simulink model "CHEM_FULL_BENCHMARK"  (R2019a)
settings: Solver=FixedStepAuto  StartTime=0.0  StopTime=app.SimuTime  FixedStep=Te  RelTol=1e-3  EnableMultiTasking=on
values from neighbouring files (symbols this model uses):
  A1 = 0.0154    [INIT_FULL.m]    (also in run.m)
  A2 = 0.0154    [INIT_FULL.m]    (also in run.m)
  app = interface    [INIT_FULL.m]    (also in run.m)
  Cvb = 1.5938*1e-4    (= 0.00015938)    [INIT_FULL.m]    (also in run.m)
  Cvo = 1.59640*1e-4    (= 0.00015964)    [INIT_FULL.m]    (also in run.m)
  g = 9.81    [INIT_FULL.m]    (also in run.m)
  h1c = 0.5    [INIT_FULL.m]    (also in run.m)
  h1c_0 = 0    [INIT_FULL.m]    (also in run.m)
  h1max = 0.6    [INIT_FULL.m]    (also in run.m)
  h2c_0 = 0    [INIT_FULL.m]    (also in Variables_Update.m = app.InitialwaterlevelinT206EditField.Value; run.m)
  h2c_max = 0.11    [INIT_FULL.m]    (also in run.m)
  h2c_min = 0.09    [INIT_FULL.m]    (also in run.m)
  h2max = 0.6    [INIT_FULL.m]    (also in run.m)
  Ki = 5*1e-6    (= 5e-06)    [INIT_FULL.m]    (also in run.m)
  Kp = 1e-3    (= 0.001)    [INIT_FULL.m]    (also in run.m)
  Patm = 101325    [INIT_FULL.m]    (also in run.m)
  Qf1 = 1e-4    (= 0.0001)    [INIT_FULL.m]    (also in Variables_Update.m = app.FlowleakfromT1m3sEditField.Value; run.m)
  Qf2 = 1e-4    (= 0.0001)    [INIT_FULL.m]    (also in Variables_Update.m = app.FlowleakfromT2m3sEditField.Value; run.m)
  Qof1 = 1e-4    (= 0.0001)    [INIT_FULL.m]    (also in Variables_Update.m = app.OverflowrateinT1m3sEditField.Value; run.m)
  Qpmax = 1e-2    (= 0.01)    [INIT_FULL.m]    (also in run.m)
  rate_noise_mQp = 0.01*1e-5    (= 1e-07)    [INIT_FULL.m]    (also in run.m)
  rate_noise_mUp = 0.01*1e-5    (= 1e-07)    [INIT_FULL.m]    (also in run.m)
  rate_noise_my1 = 0.5*0.001    (= 0.0005)    [INIT_FULL.m]    (also in run.m)
  rate_noise_my2 = 0.3*0.001    (= 0.0003)    [INIT_FULL.m]    (also in run.m)
  ro = 1000    [INIT_FULL.m]    (also in run.m)
  seed = randi(10000000)    [INIT_FULL.m]    (also in run.m)
  Te = 1    [INIT_FULL.m]    (also in run.m)
  yo = 0    [INIT_FULL.m]    (also in run.m)
(part 5 of 12)

== system CHEM_FULL_BENCHMARK/T1 hidden long theft/Process/Subsystem3 ==
  note: SIMULATION OF THE VALVE Vo
  note: sign(y2-y0)
  U0 : Inport
  y2 : Inport  Port=2
  y0 : Inport  Port=3
  Abs : Abs  SaturateOnIntegerOverflow=on
  Consumer flow : Scope
  Gain : Gain  Gain=Cvo  SaturateOnIntegerOverflow=on  OutDataTypeStr=Inherit: Same as input  ParamDataTypeStr=Inherit: Same as input
  Math Function : Math  Operator=sqrt  SaturateOnIntegerOverflow=on
  Product1 : Product  SaturateOnIntegerOverflow=on  InputSameDT=on  OutDataTypeStr=Inherit: Same as first input
  Product2 : Product  SaturateOnIntegerOverflow=on  InputSameDT=on  OutDataTypeStr=Inherit: Same as first input
  Sign(x1-x2) : Signum
  Sum : Sum  Inputs=+-  SaturateOnIntegerOverflow=on  InputSameDT=on  OutDataTypeStr=Inherit: Same as first input
  Qv0 : Outport  InitialOutput=0
  wires:
  Product1/1 -> Consumer flow/1, Qv0/1
  Product2/1 -> Gain/1
  y0/1 -> Sum/2
  y2/1 -> Sum/1
  Sign(x1-x2)/1 -> Product2/1
  Math Function/1 -> Product2/2
  Abs/1 -> Math Function/1
  Sum/1 -> Abs/1, Sign(x1-x2)/1
  Gain/1 -> Product1/1
  U0/1 -> Product1/2

== system CHEM_FULL_BENCHMARK/T1 hidden long theft/Process/Subsystem4 ==
  note: SIMULATION OF THE CONTROLLER ON-OFF
  note: Ub
  note: my2
  In2 : Inport
  ON-OFF : Relay  OnSwitchValue=h2c_max  OffSwitchValue=h2c_min  OnOutputValue=0  OffOutputValue=1
  Out5 : Outport  InitialOutput=0
  wires:
  In2/1 -> ON-OFF/1
  ON-OFF/1 -> Out5/1

== system CHEM_FULL_BENCHMARK/T1 hidden long theft/Process/Subsystem5 ==
  note: SIMULATION OF THE SENSOR P1
  note: Faultless mode
  note: Faulty mode
  y1 : Inport
  Clock2 : Clock
  Commande vanne 2 : ManualSwitch
  Constant : Constant  Value=Patm
  Constant1 : Constant  Value=0
  Gain : Gain  Gain=ro*g
  Sum : Sum
  Sum6 : Sum  SaturateOnIntegerOverflow=on  InputSameDT=on  OutDataTypeStr=Inherit: Same as first input
  Switch1 : Switch  Threshold=40  SaturateOnIntegerOverflow=on  InputSameDT=on
  Switch4 : Switch  Threshold=120  SaturateOnIntegerOverflow=on  InputSameDT=on
  my1 noise : UniformRandomNumber  Minimum=-rate_noise_my1  Maximum=rate_noise_my1  Seed=seed  SampleTime=0
  mP1 : Outport  InitialOutput=0
  wires:
  Clock2/1 -> Switch1/2, Switch4/2
  Constant1/1 -> Switch1/1
  Switch1/1 -> Switch4/3
  Switch4/1 -> Commande vanne 2/2
  y1/1 -> Gain/1
  Gain/1 -> Sum/1
  Sum/1 -> Switch1/3, Commande vanne 2/1, Switch4/1
  Constant/1 -> Sum/2
  my1 noise/1 -> Sum6/2
  Sum6/1 -> mP1/1
  Commande vanne 2/1 -> Sum6/1

== system CHEM_FULL_BENCHMARK/T1 hidden long theft/Process/Subsystem6 ==
  note: SIMULATION OF THE PUMP
  note: Up
  note: Qp
  note: Qp
  note: Faultless mode
  note: Faulty mode
  Up : Inport
  Clock2 : Clock
  Commande vanne 2 : ManualSwitch
  Constant1 : Constant  Value=0
  Saturation2 : Saturate  UpperLimit=Qpmax  LowerLimit=0  LinearizeAsGain=off
  Switch1 : Switch  Threshold=40  SaturateOnIntegerOverflow=on  InputSameDT=on
  Switch4 : Switch  Threshold=80  SaturateOnIntegerOverflow=on  InputSameDT=on
  mUp : Outport  InitialOutput=0
  wires:
  Clock2/1 -> Switch1/2, Switch4/2
  Up/1 -> Switch1/3, Switch4/1, Saturation2/1
  Constant1/1 -> Switch1/1
  Switch1/1 -> Switch4/3
  Commande vanne 2/1 -> mUp/1
  Saturation2/1 -> Commande vanne 2/1
  Switch4/1 -> Commande vanne 2/2

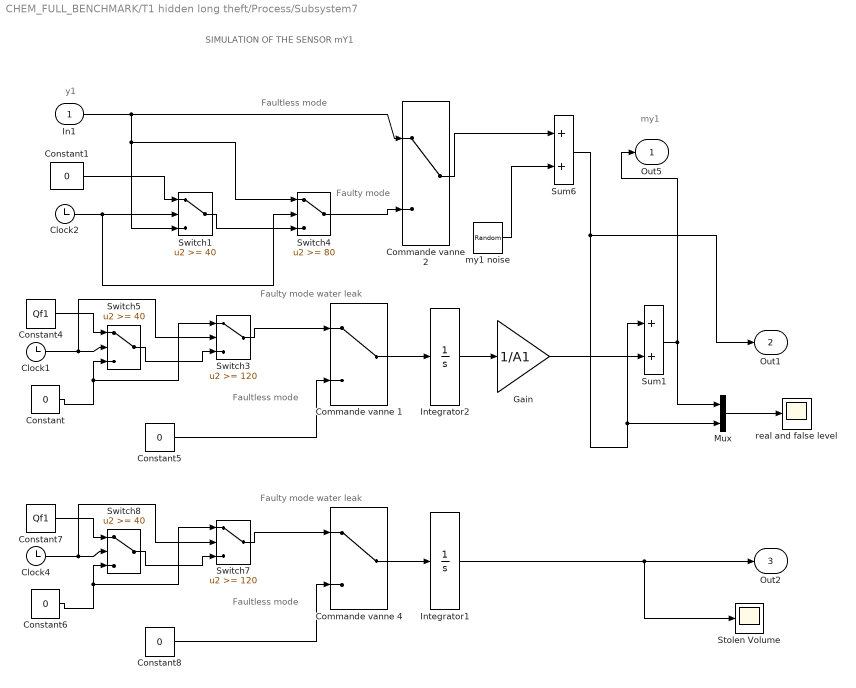
== system CHEM_FULL_BENCHMARK/T1 hidden long theft/Process/Subsystem7 ==
  note: SIMULATION OF THE SENSOR mY1
  note: y1
  note: my1
  note: Faultless mode
  note: Faulty mode
  note: Faultless mode
  note: Faulty mode
      | water leak
  note: Faultless mode
  note: Faulty mode
      | water leak
  In1 : Inport
  Clock1 : Clock
  Clock2 : Clock
  Clock4 : Clock
  Commande vanne 1 : ManualSwitch
  Commande vanne 2 : ManualSwitch
  Commande vanne 4 : ManualSwitch
  Constant{,1,5..6,8} (5 alike) : Constant  Value=0
  Constant4 : Constant  Value=Qf1
  Constant7 : Constant  Value=Qf1
  Gain : Gain  Gain=1/A1  SaturateOnIntegerOverflow=on  OutDataTypeStr=Inherit: Same as input  ParamDataTypeStr=Inherit: Same as input
  Integrator1 : Integrator
  Integrator2 : Integrator
  Mux : Mux  Inputs=2
  Stolen Volume : Scope
  Sum1 : Sum  SaturateOnIntegerOverflow=on  InputSameDT=on  OutDataTypeStr=Inherit: Same as first input
  Sum6 : Sum  SaturateOnIntegerOverflow=on  InputSameDT=on  OutDataTypeStr=Inherit: Same as first input
  Switch1 : Switch  Threshold=40  SaturateOnIntegerOverflow=on  InputSameDT=on
  Switch3 : Switch  Threshold=120  SaturateOnIntegerOverflow=on  InputSameDT=on
  Switch4 : Switch  Threshold=80  SaturateOnIntegerOverflow=on  InputSameDT=on
  Switch5 : Switch  Threshold=40  SaturateOnIntegerOverflow=on  InputSameDT=on
  Switch7 : Switch  Threshold=120  SaturateOnIntegerOverflow=on  InputSameDT=on
  Switch8 : Switch  Threshold=40  SaturateOnIntegerOverflow=on  InputSameDT=on
  my1 noise : UniformRandomNumber  Minimum=-rate_noise_my1  Maximum=rate_noise_my1  Seed=seed  SampleTime=0
  "real and false level " : Scope
  Out5 : Outport  InitialOutput=0
  Out1 : Outport  Port=2  InitialOutput=0
  Out2 : Outport  Port=3  InitialOutput=0
  wires:
  Clock2/1 -> Switch1/2, Switch4/2
  Constant1/1 -> Switch1/1
  Switch1/1 -> Switch4/3
  Switch4/1 -> Commande vanne 2/2
  In1/1 -> Switch1/3, Switch4/1, Commande vanne 2/1
  Commande vanne 2/1 -> Sum6/1
  my1 noise/1 -> Sum6/2
  Sum6/1 -> Out1/1, Mux/2, Sum1/1
  Clock1/1 -> Switch5/2, Switch3/2
  Constant4/1 -> Switch5/1
  Constant/1 -> Switch5/3, Switch3/1
  Switch5/1 -> Switch3/3
  Switch3/1 -> Commande vanne 1/1
  Constant5/1 -> Commande vanne 1/2
  Integrator2/1 -> Gain/1
  Mux/1 -> "real and false level "/1
  Commande vanne 1/1 -> Integrator2/1
  Gain/1 -> Sum1/2
  Clock4/1 -> Switch8/2, Switch7/2
  Constant7/1 -> Switch8/1
  Constant6/1 -> Switch8/3, Switch7/1
  Switch8/1 -> Switch7/3
  Switch7/1 -> Commande vanne 4/1
  Constant8/1 -> Commande vanne 4/2
  Integrator1/1 -> Stolen Volume/1, Out2/1
  Commande vanne 4/1 -> Integrator1/1
  Sum1/1 -> Mux/1, Out5/1

== system CHEM_FULL_BENCHMARK/T1 hidden long theft/Process/Subsystem8 ==
  note: SIMULATION OF TANK T2
  note: Faultless mode
  note: Faulty mode
      | water leak
  Qvo : Inport
  Qvb : Inport  Port=2
  Clock2 : Clock
  Commande vanne 2 : ManualSwitch  CurrentSetting=0
  Constant : Constant  Value=0
  Constant1 : Constant  Value=Qf2
  Constant2 : Constant  Value=0
  Gain : Gain  Gain=1/A2  SaturateOnIntegerOverflow=on  OutDataTypeStr=Inherit: Same as input  ParamDataTypeStr=Inherit: Same as input
  Integrator2 : Integrator  InitialCondition=h2c_0
  Saturation1 : Saturate  UpperLimit=h2max  LowerLimit=0  LinearizeAsGain=off
  Sum2 : Sum  Inputs=-+-  SaturateOnIntegerOverflow=on  InputSameDT=on  OutDataTypeStr=Inherit: Same as first input
  Switch1 : Switch  Threshold=120  SaturateOnIntegerOverflow=on  InputSameDT=on
  Switch4 : Switch  Threshold=40  SaturateOnIntegerOverflow=on  InputSameDT=on
  y2 : Outport  InitialOutput=0
  wires:
  Qvb/1 -> Sum2/2
  Qvo/1 -> Sum2/1
  Sum2/1 -> Gain/1
  Gain/1 -> Integrator2/1
  Clock2/1 -> Switch4/2, Switch1/2
  Constant1/1 -> Switch4/1
  Constant/1 -> Switch4/3, Switch1/1
  Switch4/1 -> Switch1/3
  Commande vanne 2/1 -> Sum2/3
  Switch1/1 -> Commande vanne 2/1
  Constant2/1 -> Commande vanne 2/2
  Integrator2/1 -> Saturation1/1
  Saturation1/1 -> y2/1

== system CHEM_FULL_BENCHMARK/T1 hidden long theft/Process/Subsystem9 ==
  Subsystem1 : Subsystem
      mask Display: disp('Set \nvalve  V2')
  Subsystem12 : Subsystem
      mask Display: disp('Set\n point h1c')
  Out3 : Outport  InitialOutput=0
  Out1 : Outport  Port=2  InitialOutput=0
  wires:
  Subsystem1/1(Out1) -> Out1/1
  Subsystem12/1(Out1) -> Out3/1

== system CHEM_FULL_BENCHMARK/T1 hidden short theft/Process/Subsystem1 ==
  note: TANK T1 SIMULATION
  note: Qf1
  note: Faultless mode
  note: Faulty mode
      | water leak
  Qp : Inport
  Qvb : Inport  Port=2
  Clock2 : Clock
  Constant : Constant  Value=0
  Constant2 : Constant  Value=0
  Gain : Gain  Gain=1/A1  SaturateOnIntegerOverflow=on  OutDataTypeStr=Inherit: Same as input  ParamDataTypeStr=Inherit: Same as input
  Integrator2 : Integrator  InitialCondition=h1c_0
  Saturation1 : Saturate  UpperLimit=h1max  LowerLimit=0  LinearizeAsGain=off
  Selector : ManualSwitch
  Sum2 : Sum  Inputs=+--  SaturateOnIntegerOverflow=on  InputSameDT=on  OutDataTypeStr=Inherit: Same as first input
  Switch1 : Switch  Threshold=80  SaturateOnIntegerOverflow=on  InputSameDT=on
  Switch4 : Switch  Threshold=40  SaturateOnIntegerOverflow=on  InputSameDT=on
  flow leak : Constant  Value=Qf1
  y1 : Outport  InitialOutput=0
  wires:
  Gain/1 -> Integrator2/1
  Sum2/1 -> Gain/1
  Qp/1 -> Sum2/1
  Qvb/1 -> Sum2/2
  Clock2/1 -> Switch4/2, Switch1/2
  flow leak/1 -> Switch4/1
  Constant/1 -> Switch4/3, Switch1/1
  Switch4/1 -> Switch1/3
  Selector/1 -> Sum2/3
  Switch1/1 -> Selector/1
  Constant2/1 -> Selector/2
  Integrator2/1 -> Saturation1/1
  Saturation1/1 -> y1/1

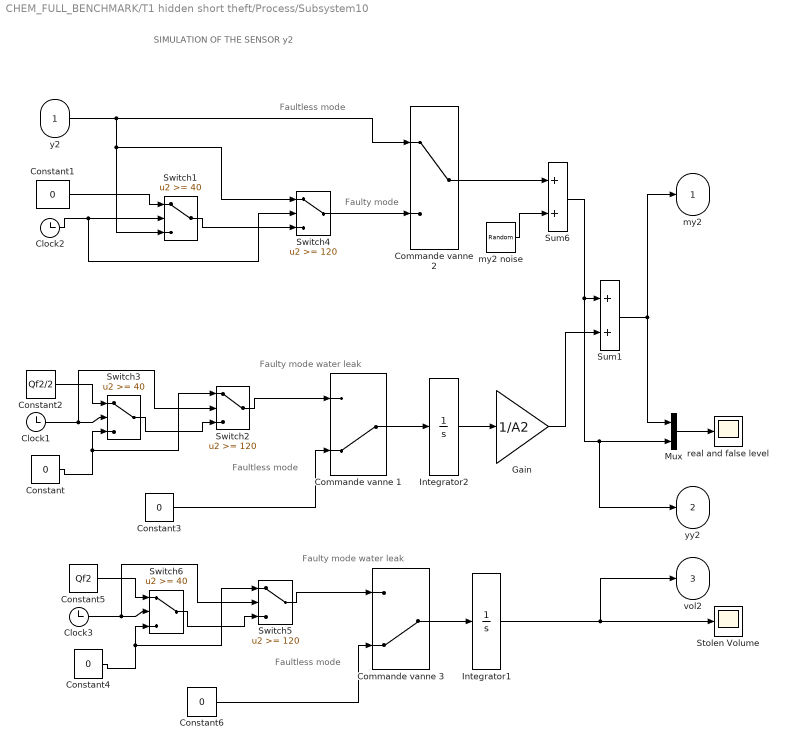
== system CHEM_FULL_BENCHMARK/T1 hidden short theft/Process/Subsystem10 ==
  note: SIMULATION OF THE SENSOR y2
  note: Faultless mode
  note: Faulty mode
  note: Faultless mode
  note: Faulty mode
      | water leak
  note: Faultless mode
  note: Faulty mode
      | water leak
  y2 : Inport
  Clock1 : Clock
  Clock2 : Clock
  Clock3 : Clock
  Commande vanne 1 : ManualSwitch  CurrentSetting=0
  Commande vanne 2 : ManualSwitch
  Commande vanne 3 : ManualSwitch  CurrentSetting=0
  Constant{,1,3..4,6} (5 alike) : Constant  Value=0
  Constant2 : Constant  Value=Qf2/2
  Constant5 : Constant  Value=Qf2
  Gain : Gain  Gain=1/A2  SaturateOnIntegerOverflow=on  OutDataTypeStr=Inherit: Same as input  ParamDataTypeStr=Inherit: Same as input
  Integrator1 : Integrator
  Integrator2 : Integrator
  Mux : Mux  Inputs=2
  Stolen Volume : Scope
  Sum1 : Sum  SaturateOnIntegerOverflow=on  InputSameDT=on  OutDataTypeStr=Inherit: Same as first input
  Sum6 : Sum  SaturateOnIntegerOverflow=on  InputSameDT=on  OutDataTypeStr=Inherit: Same as first input
  Switch1 : Switch  Threshold=40  SaturateOnIntegerOverflow=on  InputSameDT=on
  Switch2 : Switch  Threshold=120  SaturateOnIntegerOverflow=on  InputSameDT=on
  Switch3 : Switch  Threshold=40  SaturateOnIntegerOverflow=on  InputSameDT=on
  Switch4 : Switch  Threshold=120  SaturateOnIntegerOverflow=on  InputSameDT=on
  Switch5 : Switch  Threshold=120  SaturateOnIntegerOverflow=on  InputSameDT=on
  Switch6 : Switch  Threshold=40  SaturateOnIntegerOverflow=on  InputSameDT=on
  my2 noise : UniformRandomNumber  Minimum=-rate_noise_my2  Maximum=rate_noise_my2  Seed=seed  SampleTime=0
  "real and false level " : Scope
  my2 : Outport  InitialOutput=0
  yy2 : Outport  Port=2  InitialOutput=0
  vol2 : Outport  Port=3  InitialOutput=0
  wires:
  my2 noise/1 -> Sum6/2
  Commande vanne 2/1 -> Sum6/1
  y2/1 -> Commande vanne 2/1, Switch1/3, Switch4/1
  Switch4/1 -> Commande vanne 2/2
  Switch1/1 -> Switch4/3
  Constant1/1 -> Switch1/1
  Clock2/1 -> Switch4/2, Switch1/2
  Clock1/1 -> Switch3/2, Switch2/2
  Constant2/1 -> Switch3/1
  Constant/1 -> Switch3/3, Switch2/1
  Switch3/1 -> Switch2/3
  Switch2/1 -> Commande vanne 1/1
  Constant3/1 -> Commande vanne 1/2
  Sum6/1 -> yy2/1, Mux/2, Sum1/1
  Sum1/1 -> Mux/1, my2/1
  Integrator2/1 -> Gain/1
  Mux/1 -> "real and false level "/1
  Commande vanne 1/1 -> Integrator2/1
  Gain/1 -> Sum1/2
  Clock3/1 -> Switch6/2, Switch5/2
  Constant5/1 -> Switch6/1
  Constant4/1 -> Switch6/3, Switch5/1
  Switch6/1 -> Switch5/3
  Switch5/1 -> Commande vanne 3/1
  Constant6/1 -> Commande vanne 3/2
  Integrator1/1 -> vol2/1, Stolen Volume/1
  Commande vanne 3/1 -> Integrator1/1

== system CHEM_FULL_BENCHMARK/T1 hidden short theft/Process/Subsystem11 ==
  note: Faultless mode
  note: Faulty mode
  note: Up
  note: SIMULATION OF THE DIGITAL PI CONTROLLER
  h1c : Inport
  my1 : Inport  Port=2
  Clock2 : Clock
  Commande vanne 2 : ManualSwitch
  Constant1 : Constant  Value=0
  Digital PIController : DiscreteTransferFcn  Numerator=[(Ki*Te+Kp) -Kp]  Denominator=[1 -1]
  Sum : Sum  Inputs=+-  SaturateOnIntegerOverflow=on  InputSameDT=on  OutDataTypeStr=Inherit: Same as first input
  Switch1 : Switch  Threshold=40  SaturateOnIntegerOverflow=on  InputSameDT=on
  Switch4 : Switch  Threshold=120  SaturateOnIntegerOverflow=on  InputSameDT=on
  Zero-Order Hold4 : ZeroOrderHold  SampleTime=-1
  mUp : Outport  InitialOutput=0
  wires:
  Switch4/1 -> Commande vanne 2/2
  Commande vanne 2/1 -> mUp/1
  Digital PIController/1 -> Switch1/3, Switch4/1, Commande vanne 2/1
  Switch1/1 -> Switch4/3
  Constant1/1 -> Switch1/1
  Clock2/1 -> Switch4/2, Switch1/2
  h1c/1 -> Sum/1
  my1/1 -> Sum/2
  Zero-Order Hold4/1 -> Digital PIController/1
  Sum/1 -> Zero-Order Hold4/1

== system CHEM_FULL_BENCHMARK/T1 hidden short theft/Process/Subsystem12 ==
  note: SIMULATION OF THE SENSOR Ub
  note: Faultless mode
  note: Faulty mode
  Ub : Inport
  Clock2 : Clock
  Commande vanne 2 : ManualSwitch
  Constant1 : Constant  Value=0
  Switch1 : Switch  Threshold=40  SaturateOnIntegerOverflow=on  InputSameDT=on
  Switch4 : Switch  Threshold=120  SaturateOnIntegerOverflow=on  InputSameDT=on
  mUb : Outport  InitialOutput=0
  wires:
  Clock2/1 -> Switch1/2, Switch4/2
  Constant1/1 -> Switch1/1
  Switch1/1 -> Switch4/3
  Switch4/1 -> Commande vanne 2/2
  Ub/1 -> Commande vanne 2/1, Switch1/3, Switch4/1
  Commande vanne 2/1 -> mUb/1

== system CHEM_FULL_BENCHMARK/T1 hidden short theft/Process/Subsystem13 ==
  note: SIMULATION OF THE SENSOR Up
  note: Faultless mode
  note: Faulty mode
  Up : Inport
  Clock2 : Clock
  Commande vanne 2 : ManualSwitch
  Constant1 : Constant  Value=0
  Sum1 : Sum  SaturateOnIntegerOverflow=on  InputSameDT=on  OutDataTypeStr=Inherit: Same as first input
  Switch1 : Switch  Threshold=40  SaturateOnIntegerOverflow=on  InputSameDT=on
  Switch4 : Switch  Threshold=80  SaturateOnIntegerOverflow=on  InputSameDT=on
  mUp noise : UniformRandomNumber  Minimum=-rate_noise_mUp  Maximum=rate_noise_mUp  Seed=seed  SampleTime=0
  mUp : Outport  InitialOutput=0
  wires:
  Up/1 -> Commande vanne 2/1, Switch1/3, Switch4/1
  Clock2/1 -> Switch1/2, Switch4/2
  Constant1/1 -> Switch1/1
  Switch1/1 -> Switch4/3
  Switch4/1 -> Commande vanne 2/2
  Sum1/1 -> mUp/1
  mUp noise/1 -> Sum1/2
  Commande vanne 2/1 -> Sum1/1

== system CHEM_FULL_BENCHMARK/T1 hidden short theft/Process/Subsystem14 ==
  note: SIMULATION OF THE SENSOR Qp
  note: Faultless mode
  note: Faulty mode
  Qp : Inport
  Clock2 : Clock
  Commande vanne 2 : ManualSwitch
  Constant1 : Constant  Value=0
  Sum6 : Sum  SaturateOnIntegerOverflow=on  InputSameDT=on  OutDataTypeStr=Inherit: Same as first input
  Switch1 : Switch  Threshold=40  SaturateOnIntegerOverflow=on  InputSameDT=on
  Switch4 : Switch  Threshold=80  SaturateOnIntegerOverflow=on  InputSameDT=on
  mQp noise : UniformRandomNumber  Minimum=-rate_noise_mQp  Maximum=rate_noise_mQp  Seed=seed  SampleTime=0
  mQp : Outport  InitialOutput=0
  wires:
  Sum6/1 -> mQp/1
  Clock2/1 -> Switch1/2, Switch4/2
  Constant1/1 -> Switch1/1
  Switch1/1 -> Switch4/3
  Qp/1 -> Commande vanne 2/1, Switch1/3, Switch4/1
  Commande vanne 2/1 -> Sum6/1
  Switch4/1 -> Commande vanne 2/2
  mQp noise/1 -> Sum6/2

== system CHEM_FULL_BENCHMARK/T1 hidden short theft/Process/Subsystem15 ==
  note: SIMULATION OF THE SENSOR P1
  note: Faultless mode
  note: Faulty mode
  y2 : Inport
  Clock2 : Clock
  Commande vanne 2 : ManualSwitch
  Constant : Constant  Value=Patm
  Constant1 : Constant  Value=0
  Gain : Gain  Gain=ro*g
  Sum : Sum
  Sum6 : Sum  SaturateOnIntegerOverflow=on  InputSameDT=on  OutDataTypeStr=Inherit: Same as first input
  Switch1 : Switch  Threshold=40  SaturateOnIntegerOverflow=on  InputSameDT=on
  Switch4 : Switch  Threshold=120  SaturateOnIntegerOverflow=on  InputSameDT=on
  my1 noise : UniformRandomNumber  Minimum=-rate_noise_my1  Maximum=rate_noise_my1  Seed=seed  SampleTime=0
  mP2 : Outport  InitialOutput=0
  wires:
  Clock2/1 -> Switch1/2, Switch4/2
  Constant1/1 -> Switch1/1
  Switch1/1 -> Switch4/3
  Switch4/1 -> Commande vanne 2/2
  y2/1 -> Gain/1
  Gain/1 -> Sum/1
  Sum/1 -> Switch1/3, Commande vanne 2/1, Switch4/1
  Constant/1 -> Sum/2
  Sum6/1 -> mP2/1
  Commande vanne 2/1 -> Sum6/1
  my1 noise/1 -> Sum6/2

== system CHEM_FULL_BENCHMARK/T1 hidden short theft/Process/Subsystem2 ==
  note: SIMULATION OF VALVE Vb
  note: sign(y1-y2)
  note: Valve fault
      | Vb=0: Valve Vb blocked closed
      | Vb1=1: Valve Vb blocked opened
  note: Faultless mode
  note: Faulty mode
  Ub : Inport
  y1 : Inport  Port=2
  y2 : Inport  Port=3
  Abs : Abs  SaturateOnIntegerOverflow=on
  Clock2 : Clock
  Commande vanne 1 : ManualSwitch
  Commande vanne 2 : ManualSwitch
  Gain : Gain  Gain=Cvb  SaturateOnIntegerOverflow=on  OutDataTypeStr=Inherit: Same as input  ParamDataTypeStr=Inherit: Same as input
  Math Function : Math  Operator=sqrt  SaturateOnIntegerOverflow=on
  Product1 : Product  SaturateOnIntegerOverflow=on  InputSameDT=on  OutDataTypeStr=Inherit: Same as first input
  Product2 : Product  SaturateOnIntegerOverflow=on  InputSameDT=on  OutDataTypeStr=Inherit: Same as first input
  Sign(x1-x2) : Signum
  Sum : Sum  Inputs=+-  SaturateOnIntegerOverflow=on  InputSameDT=on  OutDataTypeStr=Inherit: Same as first input
  Switch1 : Switch  Threshold=150  SaturateOnIntegerOverflow=on  InputSameDT=on
  Switch4 : Switch  Threshold=40  SaturateOnIntegerOverflow=on  InputSameDT=on
  Vb : Constant  Value=0
  Vb1 : Constant
  QVb : Outport  InitialOutput=0
  wires:
  Gain/1 -> Product1/1
  Product1/1 -> QVb/1
  Product2/1 -> Gain/1
  y1/1 -> Sum/1
  Sign(x1-x2)/1 -> Product2/1
  Math Function/1 -> Product2/2
  Abs/1 -> Math Function/1
  Sum/1 -> Abs/1, Sign(x1-x2)/1
  y2/1 -> Sum/2
  Vb/1 -> Commande vanne 1/1
  Vb1/1 -> Commande vanne 1/2
  Clock2/1 -> Switch4/2, Switch1/2
  Ub/1 -> Commande vanne 2/1, Switch4/3, Switch1/1
  Commande vanne 1/1 -> Switch4/1
  Switch1/1 -> Commande vanne 2/2
  Switch4/1 -> Switch1/3
  Commande vanne 2/1 -> Product1/2

== system CHEM_FULL_BENCHMARK/T1 hidden short theft/Process/Subsystem3 ==
  note: SIMULATION OF THE VALVE Vo
  note: sign(y2-y0)
  U0 : Inport
  y2 : Inport  Port=2
  y0 : Inport  Port=3
  Abs : Abs  SaturateOnIntegerOverflow=on
  Consumer flow : Scope
  Gain : Gain  Gain=Cvo  SaturateOnIntegerOverflow=on  OutDataTypeStr=Inherit: Same as input  ParamDataTypeStr=Inherit: Same as input
  Math Function : Math  Operator=sqrt  SaturateOnIntegerOverflow=on
  Product1 : Product  SaturateOnIntegerOverflow=on  InputSameDT=on  OutDataTypeStr=Inherit: Same as first input
  Product2 : Product  SaturateOnIntegerOverflow=on  InputSameDT=on  OutDataTypeStr=Inherit: Same as first input
  Sign(x1-x2) : Signum
  Sum : Sum  Inputs=+-  SaturateOnIntegerOverflow=on  InputSameDT=on  OutDataTypeStr=Inherit: Same as first input
  Qv0 : Outport  InitialOutput=0
  wires:
  Product1/1 -> Consumer flow/1, Qv0/1
  Product2/1 -> Gain/1
  y0/1 -> Sum/2
  y2/1 -> Sum/1
  Sign(x1-x2)/1 -> Product2/1
  Math Function/1 -> Product2/2
  Abs/1 -> Math Function/1
  Sum/1 -> Abs/1, Sign(x1-x2)/1
  Gain/1 -> Product1/1
  U0/1 -> Product1/2

== system CHEM_FULL_BENCHMARK/T1 hidden short theft/Process/Subsystem4 ==
  note: SIMULATION OF THE CONTROLLER ON-OFF
  note: Ub
  note: my2
  In2 : Inport
  ON-OFF : Relay  OnSwitchValue=h2c_max  OffSwitchValue=h2c_min  OnOutputValue=0  OffOutputValue=1
  Out5 : Outport  InitialOutput=0
  wires:
  In2/1 -> ON-OFF/1
  ON-OFF/1 -> Out5/1

== system CHEM_FULL_BENCHMARK/T1 hidden short theft/Process/Subsystem5 ==
  note: SIMULATION OF THE SENSOR P1
  note: Faultless mode
  note: Faulty mode
  y1 : Inport
  Clock2 : Clock
  Commande vanne 2 : ManualSwitch
  Constant : Constant  Value=Patm
  Constant1 : Constant  Value=0
  Gain : Gain  Gain=ro*g
  Sum : Sum
  Sum6 : Sum  SaturateOnIntegerOverflow=on  InputSameDT=on  OutDataTypeStr=Inherit: Same as first input
  Switch1 : Switch  Threshold=40  SaturateOnIntegerOverflow=on  InputSameDT=on
  Switch4 : Switch  Threshold=120  SaturateOnIntegerOverflow=on  InputSameDT=on
  my1 noise : UniformRandomNumber  Minimum=-rate_noise_my1  Maximum=rate_noise_my1  Seed=seed  SampleTime=0
  mP1 : Outport  InitialOutput=0
  wires:
  Clock2/1 -> Switch1/2, Switch4/2
  Constant1/1 -> Switch1/1
  Switch1/1 -> Switch4/3
  Switch4/1 -> Commande vanne 2/2
  y1/1 -> Gain/1
  Gain/1 -> Sum/1
  Sum/1 -> Switch1/3, Commande vanne 2/1, Switch4/1
  Constant/1 -> Sum/2
  my1 noise/1 -> Sum6/2
  Sum6/1 -> mP1/1
  Commande vanne 2/1 -> Sum6/1

== system CHEM_FULL_BENCHMARK/T1 hidden short theft/Process/Subsystem6 ==
  note: SIMULATION OF THE PUMP
  note: Up
  note: Qp
  note: Qp
  note: Faultless mode
  note: Faulty mode
  Up : Inport
  Clock2 : Clock
  Commande vanne 2 : ManualSwitch
  Constant1 : Constant  Value=0
  Saturation2 : Saturate  UpperLimit=Qpmax  LowerLimit=0  LinearizeAsGain=off
  Switch1 : Switch  Threshold=40  SaturateOnIntegerOverflow=on  InputSameDT=on
  Switch4 : Switch  Threshold=80  SaturateOnIntegerOverflow=on  InputSameDT=on
  mUp : Outport  InitialOutput=0
  wires:
  Clock2/1 -> Switch1/2, Switch4/2
  Up/1 -> Switch1/3, Switch4/1, Saturation2/1
  Constant1/1 -> Switch1/1
  Switch1/1 -> Switch4/3
  Commande vanne 2/1 -> mUp/1
  Saturation2/1 -> Commande vanne 2/1
  Switch4/1 -> Commande vanne 2/2

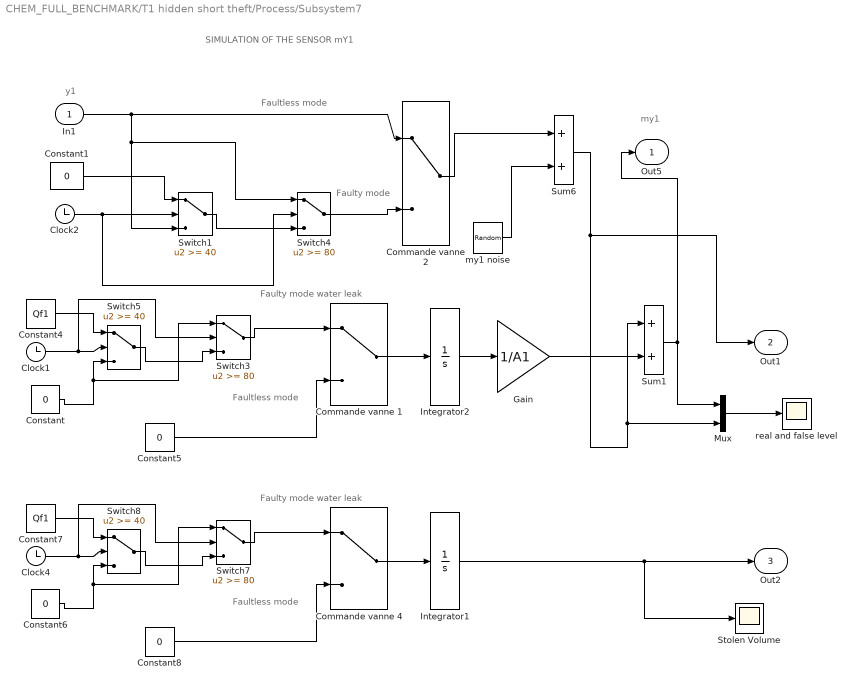
== system CHEM_FULL_BENCHMARK/T1 hidden short theft/Process/Subsystem7 ==
  note: SIMULATION OF THE SENSOR mY1
  note: y1
  note: my1
  note: Faultless mode
  note: Faulty mode
  note: Faultless mode
  note: Faulty mode
      | water leak
  note: Faultless mode
  note: Faulty mode
      | water leak
  In1 : Inport
  Clock1 : Clock
  Clock2 : Clock
  Clock4 : Clock
  Commande vanne 1 : ManualSwitch
  Commande vanne 2 : ManualSwitch
  Commande vanne 4 : ManualSwitch
  Constant{,1,5..6,8} (5 alike) : Constant  Value=0
  Constant4 : Constant  Value=Qf1
  Constant7 : Constant  Value=Qf1
  Gain : Gain  Gain=1/A1  SaturateOnIntegerOverflow=on  OutDataTypeStr=Inherit: Same as input  ParamDataTypeStr=Inherit: Same as input
  Integrator1 : Integrator
  Integrator2 : Integrator
  Mux : Mux  Inputs=2
  Stolen Volume : Scope
  Sum1 : Sum  SaturateOnIntegerOverflow=on  InputSameDT=on  OutDataTypeStr=Inherit: Same as first input
  Sum6 : Sum  SaturateOnIntegerOverflow=on  InputSameDT=on  OutDataTypeStr=Inherit: Same as first input
  Switch1 : Switch  Threshold=40  SaturateOnIntegerOverflow=on  InputSameDT=on
  Switch3 : Switch  Threshold=80  SaturateOnIntegerOverflow=on  InputSameDT=on
  Switch4 : Switch  Threshold=80  SaturateOnIntegerOverflow=on  InputSameDT=on
  Switch5 : Switch  Threshold=40  SaturateOnIntegerOverflow=on  InputSameDT=on
  Switch7 : Switch  Threshold=80  SaturateOnIntegerOverflow=on  InputSameDT=on
  Switch8 : Switch  Threshold=40  SaturateOnIntegerOverflow=on  InputSameDT=on
  my1 noise : UniformRandomNumber  Minimum=-rate_noise_my1  Maximum=rate_noise_my1  Seed=seed  SampleTime=0
  "real and false level " : Scope
  Out5 : Outport  InitialOutput=0
  Out1 : Outport  Port=2  InitialOutput=0
  Out2 : Outport  Port=3  InitialOutput=0
  wires:
  Clock2/1 -> Switch1/2, Switch4/2
  Constant1/1 -> Switch1/1
  Switch1/1 -> Switch4/3
  Switch4/1 -> Commande vanne 2/2
  In1/1 -> Switch1/3, Switch4/1, Commande vanne 2/1
  Commande vanne 2/1 -> Sum6/1
  my1 noise/1 -> Sum6/2
  Sum6/1 -> Out1/1, Mux/2, Sum1/1
  Clock1/1 -> Switch5/2, Switch3/2
  Constant4/1 -> Switch5/1
  Constant/1 -> Switch5/3, Switch3/1
  Switch5/1 -> Switch3/3
  Switch3/1 -> Commande vanne 1/1
  Constant5/1 -> Commande vanne 1/2
  Integrator2/1 -> Gain/1
  Mux/1 -> "real and false level "/1
  Commande vanne 1/1 -> Integrator2/1
  Gain/1 -> Sum1/2
  Clock4/1 -> Switch8/2, Switch7/2
  Constant7/1 -> Switch8/1
  Constant6/1 -> Switch8/3, Switch7/1
  Switch8/1 -> Switch7/3
  Switch7/1 -> Commande vanne 4/1
  Constant8/1 -> Commande vanne 4/2
  Integrator1/1 -> Stolen Volume/1, Out2/1
  Commande vanne 4/1 -> Integrator1/1
  Sum1/1 -> Mux/1, Out5/1

== system CHEM_FULL_BENCHMARK/T1 hidden short theft/Process/Subsystem8 ==
  note: SIMULATION OF TANK T2
  note: Faultless mode
  note: Faulty mode
      | water leak
  Qvo : Inport
  Qvb : Inport  Port=2
  Clock2 : Clock
  Commande vanne 2 : ManualSwitch  CurrentSetting=0
  Constant : Constant  Value=0
  Constant1 : Constant  Value=Qf2
  Constant2 : Constant  Value=0
  Gain : Gain  Gain=1/A2  SaturateOnIntegerOverflow=on  OutDataTypeStr=Inherit: Same as input  ParamDataTypeStr=Inherit: Same as input
  Integrator2 : Integrator  InitialCondition=h2c_0
  Saturation1 : Saturate  UpperLimit=h2max  LowerLimit=0  LinearizeAsGain=off
  Sum2 : Sum  Inputs=-+-  SaturateOnIntegerOverflow=on  InputSameDT=on  OutDataTypeStr=Inherit: Same as first input
  Switch1 : Switch  Threshold=120  SaturateOnIntegerOverflow=on  InputSameDT=on
  Switch4 : Switch  Threshold=40  SaturateOnIntegerOverflow=on  InputSameDT=on
  y2 : Outport  InitialOutput=0
  wires:
  Qvb/1 -> Sum2/2
  Qvo/1 -> Sum2/1
  Sum2/1 -> Gain/1
  Gain/1 -> Integrator2/1
  Clock2/1 -> Switch4/2, Switch1/2
  Constant1/1 -> Switch4/1
  Constant/1 -> Switch4/3, Switch1/1
  Switch4/1 -> Switch1/3
  Commande vanne 2/1 -> Sum2/3
  Switch1/1 -> Commande vanne 2/1
  Constant2/1 -> Commande vanne 2/2
  Integrator2/1 -> Saturation1/1
  Saturation1/1 -> y2/1

== system CHEM_FULL_BENCHMARK/T1 hidden short theft/Process/Subsystem9 ==
  Subsystem1 : Subsystem
      mask Display: disp('Set \nvalve  V2')
  Subsystem12 : Subsystem
      mask Display: disp('Set\n point h1c')
  Out3 : Outport  InitialOutput=0
  Out1 : Outport  Port=2  InitialOutput=0
  wires:
  Subsystem1/1(Out1) -> Out1/1
  Subsystem12/1(Out1) -> Out3/1

== system CHEM_FULL_BENCHMARK/T1 semi hidden long theft/Process/Subsystem1 ==
  note: TANK T1 SIMULATION
  note: Qf1
  note: Faultless mode
  note: Faulty mode
      | water leak
  Qp : Inport
  Qvb : Inport  Port=2
  Clock2 : Clock
  Constant : Constant  Value=0
  Constant2 : Constant  Value=0
  Gain : Gain  Gain=1/A1  SaturateOnIntegerOverflow=on  OutDataTypeStr=Inherit: Same as input  ParamDataTypeStr=Inherit: Same as input
  Integrator2 : Integrator  InitialCondition=h1c_0
  Saturation1 : Saturate  UpperLimit=h1max  LowerLimit=0  LinearizeAsGain=off
  Selector : ManualSwitch
  Sum2 : Sum  Inputs=+--  SaturateOnIntegerOverflow=on  InputSameDT=on  OutDataTypeStr=Inherit: Same as first input
  Switch1 : Switch  Threshold=120  SaturateOnIntegerOverflow=on  InputSameDT=on
  Switch4 : Switch  Threshold=40  SaturateOnIntegerOverflow=on  InputSameDT=on
  flow leak : Constant  Value=Qf1
  y1 : Outport  InitialOutput=0
  wires:
  Gain/1 -> Integrator2/1
  Sum2/1 -> Gain/1
  Qp/1 -> Sum2/1
  Qvb/1 -> Sum2/2
  Clock2/1 -> Switch4/2, Switch1/2
  flow leak/1 -> Switch4/1
  Constant/1 -> Switch4/3, Switch1/1
  Switch4/1 -> Switch1/3
  Selector/1 -> Sum2/3
  Switch1/1 -> Selector/1
  Constant2/1 -> Selector/2
  Integrator2/1 -> Saturation1/1
  Saturation1/1 -> y1/1

== system CHEM_FULL_BENCHMARK/T1 semi hidden long theft/Process/Subsystem10 ==
  note: SIMULATION OF THE SENSOR y2
  note: Faultless mode
  note: Faulty mode
  note: Faultless mode
  note: Faulty mode
      | water leak
  note: Faultless mode
  note: Faulty mode
      | water leak
  y2 : Inport
  Clock1 : Clock
  Clock2 : Clock
  Clock3 : Clock
  Commande vanne 1 : ManualSwitch  CurrentSetting=0
  Commande vanne 2 : ManualSwitch
  Commande vanne 3 : ManualSwitch  CurrentSetting=0
  Constant{,1,3..4,6} (5 alike) : Constant  Value=0
  Constant2 : Constant  Value=Qf2/2
  Constant5 : Constant  Value=Qf2
  Gain : Gain  Gain=1/A2  SaturateOnIntegerOverflow=on  OutDataTypeStr=Inherit: Same as input  ParamDataTypeStr=Inherit: Same as input
  Integrator1 : Integrator
  Integrator2 : Integrator
  Mux : Mux  Inputs=2
  Stolen Volume : Scope
  Sum1 : Sum  SaturateOnIntegerOverflow=on  InputSameDT=on  OutDataTypeStr=Inherit: Same as first input
  Sum6 : Sum  SaturateOnIntegerOverflow=on  InputSameDT=on  OutDataTypeStr=Inherit: Same as first input
  Switch1 : Switch  Threshold=40  SaturateOnIntegerOverflow=on  InputSameDT=on
  Switch2 : Switch  Threshold=120  SaturateOnIntegerOverflow=on  InputSameDT=on
  Switch3 : Switch  Threshold=40  SaturateOnIntegerOverflow=on  InputSameDT=on
  Switch4 : Switch  Threshold=120  SaturateOnIntegerOverflow=on  InputSameDT=on
  Switch5 : Switch  Threshold=120  SaturateOnIntegerOverflow=on  InputSameDT=on
  Switch6 : Switch  Threshold=40  SaturateOnIntegerOverflow=on  InputSameDT=on
  my2 noise : UniformRandomNumber  Minimum=-rate_noise_my2  Maximum=rate_noise_my2  Seed=seed  SampleTime=0
  "real and false level " : Scope
  my2 : Outport  InitialOutput=0
  yy2 : Outport  Port=2  InitialOutput=0
  vol2 : Outport  Port=3  InitialOutput=0
  wires:
  my2 noise/1 -> Sum6/2
  Commande vanne 2/1 -> Sum6/1
  y2/1 -> Commande vanne 2/1, Switch1/3, Switch4/1
  Switch4/1 -> Commande vanne 2/2
  Switch1/1 -> Switch4/3
  Constant1/1 -> Switch1/1
  Clock2/1 -> Switch4/2, Switch1/2
  Clock1/1 -> Switch3/2, Switch2/2
  Constant2/1 -> Switch3/1
  Constant/1 -> Switch3/3, Switch2/1
  Switch3/1 -> Switch2/3
  Switch2/1 -> Commande vanne 1/1
  Constant3/1 -> Commande vanne 1/2
  Sum6/1 -> yy2/1, Mux/2, Sum1/1
  Sum1/1 -> Mux/1, my2/1
  Integrator2/1 -> Gain/1
  Mux/1 -> "real and false level "/1
  Commande vanne 1/1 -> Integrator2/1
  Gain/1 -> Sum1/2
  Clock3/1 -> Switch6/2, Switch5/2
  Constant5/1 -> Switch6/1
  Constant4/1 -> Switch6/3, Switch5/1
  Switch6/1 -> Switch5/3
  Switch5/1 -> Commande vanne 3/1
  Constant6/1 -> Commande vanne 3/2
  Integrator1/1 -> vol2/1, Stolen Volume/1
  Commande vanne 3/1 -> Integrator1/1

== system CHEM_FULL_BENCHMARK/T1 semi hidden long theft/Process/Subsystem11 ==
  note: Faultless mode
  note: Faulty mode
  note: Up
  note: SIMULATION OF THE DIGITAL PI CONTROLLER
  h1c : Inport
  my1 : Inport  Port=2
  Clock2 : Clock
  Commande vanne 2 : ManualSwitch
  Constant1 : Constant  Value=0
  Digital PIController : DiscreteTransferFcn  Numerator=[(Ki*Te+Kp) -Kp]  Denominator=[1 -1]
  Sum : Sum  Inputs=+-  SaturateOnIntegerOverflow=on  InputSameDT=on  OutDataTypeStr=Inherit: Same as first input
  Switch1 : Switch  Threshold=40  SaturateOnIntegerOverflow=on  InputSameDT=on
  Switch4 : Switch  Threshold=120  SaturateOnIntegerOverflow=on  InputSameDT=on
  Zero-Order Hold4 : ZeroOrderHold  SampleTime=-1
  mUp : Outport  InitialOutput=0
  wires:
  Switch4/1 -> Commande vanne 2/2
  Commande vanne 2/1 -> mUp/1
  Digital PIController/1 -> Switch1/3, Switch4/1, Commande vanne 2/1
  Switch1/1 -> Switch4/3
  Constant1/1 -> Switch1/1
  Clock2/1 -> Switch4/2, Switch1/2
  h1c/1 -> Sum/1
  my1/1 -> Sum/2
  Zero-Order Hold4/1 -> Digital PIController/1
  Sum/1 -> Zero-Order Hold4/1

== system CHEM_FULL_BENCHMARK/T1 semi hidden long theft/Process/Subsystem12 ==
  note: SIMULATION OF THE SENSOR Ub
  note: Faultless mode
  note: Faulty mode
  Ub : Inport
  Clock2 : Clock
  Commande vanne 2 : ManualSwitch
  Constant1 : Constant  Value=0
  Switch1 : Switch  Threshold=40  SaturateOnIntegerOverflow=on  InputSameDT=on
  Switch4 : Switch  Threshold=120  SaturateOnIntegerOverflow=on  InputSameDT=on
  mUb : Outport  InitialOutput=0
  wires:
  Clock2/1 -> Switch1/2, Switch4/2
  Constant1/1 -> Switch1/1
  Switch1/1 -> Switch4/3
  Switch4/1 -> Commande vanne 2/2
  Ub/1 -> Commande vanne 2/1, Switch1/3, Switch4/1
  Commande vanne 2/1 -> mUb/1

== system CHEM_FULL_BENCHMARK/T1 semi hidden long theft/Process/Subsystem13 ==
  note: SIMULATION OF THE SENSOR Up
  note: Faultless mode
  note: Faulty mode
  Up : Inport
  Clock2 : Clock
  Commande vanne 2 : ManualSwitch
  Constant1 : Constant  Value=0
  Sum1 : Sum  SaturateOnIntegerOverflow=on  InputSameDT=on  OutDataTypeStr=Inherit: Same as first input
  Switch1 : Switch  Threshold=40  SaturateOnIntegerOverflow=on  InputSameDT=on
  Switch4 : Switch  Threshold=80  SaturateOnIntegerOverflow=on  InputSameDT=on
  mUp noise : UniformRandomNumber  Minimum=-rate_noise_mUp  Maximum=rate_noise_mUp  Seed=seed  SampleTime=0
  mUp : Outport  InitialOutput=0
  wires:
  Up/1 -> Commande vanne 2/1, Switch1/3, Switch4/1
  Clock2/1 -> Switch1/2, Switch4/2
  Constant1/1 -> Switch1/1
  Switch1/1 -> Switch4/3
  Switch4/1 -> Commande vanne 2/2
  Sum1/1 -> mUp/1
  mUp noise/1 -> Sum1/2
  Commande vanne 2/1 -> Sum1/1

== system CHEM_FULL_BENCHMARK/T1 semi hidden long theft/Process/Subsystem14 ==
  note: SIMULATION OF THE SENSOR Qp
  note: Faultless mode
  note: Faulty mode
  Qp : Inport
  Clock2 : Clock
  Commande vanne 2 : ManualSwitch
  Constant1 : Constant  Value=0
  Sum6 : Sum  SaturateOnIntegerOverflow=on  InputSameDT=on  OutDataTypeStr=Inherit: Same as first input
  Switch1 : Switch  Threshold=40  SaturateOnIntegerOverflow=on  InputSameDT=on
  Switch4 : Switch  Threshold=80  SaturateOnIntegerOverflow=on  InputSameDT=on
  mQp noise : UniformRandomNumber  Minimum=-rate_noise_mQp  Maximum=rate_noise_mQp  Seed=seed  SampleTime=0
  mQp : Outport  InitialOutput=0
  wires:
  Sum6/1 -> mQp/1
  Clock2/1 -> Switch1/2, Switch4/2
  Constant1/1 -> Switch1/1
  Switch1/1 -> Switch4/3
  Qp/1 -> Commande vanne 2/1, Switch1/3, Switch4/1
  Commande vanne 2/1 -> Sum6/1
  Switch4/1 -> Commande vanne 2/2
  mQp noise/1 -> Sum6/2

== system CHEM_FULL_BENCHMARK/T1 semi hidden long theft/Process/Subsystem15 ==
  note: SIMULATION OF THE SENSOR P1
  note: Faultless mode
  note: Faulty mode
  y2 : Inport
  Clock2 : Clock
  Commande vanne 2 : ManualSwitch
  Constant : Constant  Value=Patm
  Constant1 : Constant  Value=0
  Gain : Gain  Gain=ro*g
  Sum : Sum
  Sum6 : Sum  SaturateOnIntegerOverflow=on  InputSameDT=on  OutDataTypeStr=Inherit: Same as first input
  Switch1 : Switch  Threshold=40  SaturateOnIntegerOverflow=on  InputSameDT=on
  Switch4 : Switch  Threshold=120  SaturateOnIntegerOverflow=on  InputSameDT=on
  my1 noise : UniformRandomNumber  Minimum=-rate_noise_my1  Maximum=rate_noise_my1  Seed=seed  SampleTime=0
  mP2 : Outport  InitialOutput=0
  wires:
  Clock2/1 -> Switch1/2, Switch4/2
  Constant1/1 -> Switch1/1
  Switch1/1 -> Switch4/3
  Switch4/1 -> Commande vanne 2/2
  y2/1 -> Gain/1
  Gain/1 -> Sum/1
  Sum/1 -> Switch1/3, Commande vanne 2/1, Switch4/1
  Constant/1 -> Sum/2
  Sum6/1 -> mP2/1
  Commande vanne 2/1 -> Sum6/1
  my1 noise/1 -> Sum6/2

== system CHEM_FULL_BENCHMARK/T1 semi hidden long theft/Process/Subsystem2 ==
  note: SIMULATION OF VALVE Vb
  note: sign(y1-y2)
  note: Valve fault
      | Vb=0: Valve Vb blocked closed
      | Vb1=1: Valve Vb blocked opened
  note: Faultless mode
  note: Faulty mode
  Ub : Inport
  y1 : Inport  Port=2
  y2 : Inport  Port=3
  Abs : Abs  SaturateOnIntegerOverflow=on
  Clock2 : Clock
  Commande vanne 1 : ManualSwitch
  Commande vanne 2 : ManualSwitch
  Gain : Gain  Gain=Cvb  SaturateOnIntegerOverflow=on  OutDataTypeStr=Inherit: Same as input  ParamDataTypeStr=Inherit: Same as input
  Math Function : Math  Operator=sqrt  SaturateOnIntegerOverflow=on
  Product1 : Product  SaturateOnIntegerOverflow=on  InputSameDT=on  OutDataTypeStr=Inherit: Same as first input
  Product2 : Product  SaturateOnIntegerOverflow=on  InputSameDT=on  OutDataTypeStr=Inherit: Same as first input
  Sign(x1-x2) : Signum
  Sum : Sum  Inputs=+-  SaturateOnIntegerOverflow=on  InputSameDT=on  OutDataTypeStr=Inherit: Same as first input
  Switch1 : Switch  Threshold=150  SaturateOnIntegerOverflow=on  InputSameDT=on
  Switch4 : Switch  Threshold=40  SaturateOnIntegerOverflow=on  InputSameDT=on
  Vb : Constant  Value=0
  Vb1 : Constant
  QVb : Outport  InitialOutput=0
  wires:
  Gain/1 -> Product1/1
  Product1/1 -> QVb/1
  Product2/1 -> Gain/1
  y1/1 -> Sum/1
  Sign(x1-x2)/1 -> Product2/1
  Math Function/1 -> Product2/2
  Abs/1 -> Math Function/1
  Sum/1 -> Abs/1, Sign(x1-x2)/1
  y2/1 -> Sum/2
  Vb/1 -> Commande vanne 1/1
  Vb1/1 -> Commande vanne 1/2
  Clock2/1 -> Switch4/2, Switch1/2
  Ub/1 -> Commande vanne 2/1, Switch4/3, Switch1/1
  Commande vanne 1/1 -> Switch4/1
  Switch1/1 -> Commande vanne 2/2
  Switch4/1 -> Switch1/3
  Commande vanne 2/1 -> Product1/2

== system CHEM_FULL_BENCHMARK/T1 semi hidden long theft/Process/Subsystem3 ==
  note: SIMULATION OF THE VALVE Vo
  note: sign(y2-y0)
  U0 : Inport
  y2 : Inport  Port=2
  y0 : Inport  Port=3
  Abs : Abs  SaturateOnIntegerOverflow=on
  Consumer flow : Scope
  Gain : Gain  Gain=Cvo  SaturateOnIntegerOverflow=on  OutDataTypeStr=Inherit: Same as input  ParamDataTypeStr=Inherit: Same as input
  Math Function : Math  Operator=sqrt  SaturateOnIntegerOverflow=on
  Product1 : Product  SaturateOnIntegerOverflow=on  InputSameDT=on  OutDataTypeStr=Inherit: Same as first input
  Product2 : Product  SaturateOnIntegerOverflow=on  InputSameDT=on  OutDataTypeStr=Inherit: Same as first input
  Sign(x1-x2) : Signum
  Sum : Sum  Inputs=+-  SaturateOnIntegerOverflow=on  InputSameDT=on  OutDataTypeStr=Inherit: Same as first input
  Qv0 : Outport  InitialOutput=0
  wires:
  Product1/1 -> Consumer flow/1, Qv0/1
  Product2/1 -> Gain/1
  y0/1 -> Sum/2
  y2/1 -> Sum/1
  Sign(x1-x2)/1 -> Product2/1
  Math Function/1 -> Product2/2
  Abs/1 -> Math Function/1
  Sum/1 -> Abs/1, Sign(x1-x2)/1
  Gain/1 -> Product1/1
  U0/1 -> Product1/2

== system CHEM_FULL_BENCHMARK/T1 semi hidden long theft/Process/Subsystem4 ==
  note: SIMULATION OF THE CONTROLLER ON-OFF
  note: Ub
  note: my2
  In2 : Inport
  ON-OFF : Relay  OnSwitchValue=h2c_max  OffSwitchValue=h2c_min  OnOutputValue=0  OffOutputValue=1
  Out5 : Outport  InitialOutput=0
  wires:
  In2/1 -> ON-OFF/1
  ON-OFF/1 -> Out5/1

== system CHEM_FULL_BENCHMARK/T1 semi hidden long theft/Process/Subsystem5 ==
  note: SIMULATION OF THE SENSOR P1
  note: Faultless mode
  note: Faulty mode
  y1 : Inport
  Clock2 : Clock
  Commande vanne 2 : ManualSwitch
  Constant : Constant  Value=Patm
  Constant1 : Constant  Value=0
  Gain : Gain  Gain=ro*g
  Sum : Sum
  Sum6 : Sum  SaturateOnIntegerOverflow=on  InputSameDT=on  OutDataTypeStr=Inherit: Same as first input
  Switch1 : Switch  Threshold=40  SaturateOnIntegerOverflow=on  InputSameDT=on
  Switch4 : Switch  Threshold=120  SaturateOnIntegerOverflow=on  InputSameDT=on
  my1 noise : UniformRandomNumber  Minimum=-rate_noise_my1  Maximum=rate_noise_my1  Seed=seed  SampleTime=0
  mP1 : Outport  InitialOutput=0
  wires:
  Clock2/1 -> Switch1/2, Switch4/2
  Constant1/1 -> Switch1/1
  Switch1/1 -> Switch4/3
  Switch4/1 -> Commande vanne 2/2
  y1/1 -> Gain/1
  Gain/1 -> Sum/1
  Sum/1 -> Switch1/3, Commande vanne 2/1, Switch4/1
  Constant/1 -> Sum/2
  my1 noise/1 -> Sum6/2
  Sum6/1 -> mP1/1
  Commande vanne 2/1 -> Sum6/1

== system CHEM_FULL_BENCHMARK/T1 semi hidden long theft/Process/Subsystem6 ==
  note: SIMULATION OF THE PUMP
  note: Up
  note: Qp
  note: Qp
  note: Faultless mode
  note: Faulty mode
  Up : Inport
  Clock2 : Clock
  Commande vanne 2 : ManualSwitch
  Constant1 : Constant  Value=0
  Saturation2 : Saturate  UpperLimit=Qpmax  LowerLimit=0  LinearizeAsGain=off
  Switch1 : Switch  Threshold=40  SaturateOnIntegerOverflow=on  InputSameDT=on
  Switch4 : Switch  Threshold=80  SaturateOnIntegerOverflow=on  InputSameDT=on
  mUp : Outport  InitialOutput=0
  wires:
  Clock2/1 -> Switch1/2, Switch4/2
  Up/1 -> Switch1/3, Switch4/1, Saturation2/1
  Constant1/1 -> Switch1/1
  Switch1/1 -> Switch4/3
  Commande vanne 2/1 -> mUp/1
  Saturation2/1 -> Commande vanne 2/1
  Switch4/1 -> Commande vanne 2/2

== system CHEM_FULL_BENCHMARK/T1 semi hidden long theft/Process/Subsystem7 ==
  note: SIMULATION OF THE SENSOR mY1
  note: y1
  note: my1
  note: Faultless mode
  note: Faulty mode
  note: Faultless mode
  note: Faulty mode
      | water leak
  note: Faultless mode
  note: Faulty mode
      | water leak
  In1 : Inport
  Clock1 : Clock
  Clock2 : Clock
  Clock4 : Clock
  Commande vanne 1 : ManualSwitch
  Commande vanne 2 : ManualSwitch
  Commande vanne 4 : ManualSwitch
  Constant{,1,5..6,8} (5 alike) : Constant  Value=0
  Constant4 : Constant  Value=Qf1/2
  Constant7 : Constant  Value=Qf1
  Gain : Gain  Gain=1/A1  SaturateOnIntegerOverflow=on  OutDataTypeStr=Inherit: Same as input  ParamDataTypeStr=Inherit: Same as input
  Integrator1 : Integrator
  Integrator2 : Integrator
  Mux : Mux  Inputs=2
  Stolen Volume : Scope
  Sum1 : Sum  SaturateOnIntegerOverflow=on  InputSameDT=on  OutDataTypeStr=Inherit: Same as first input
  Sum6 : Sum  SaturateOnIntegerOverflow=on  InputSameDT=on  OutDataTypeStr=Inherit: Same as first input
  Switch1 : Switch  Threshold=40  SaturateOnIntegerOverflow=on  InputSameDT=on
  Switch3 : Switch  Threshold=120  SaturateOnIntegerOverflow=on  InputSameDT=on
  Switch4 : Switch  Threshold=80  SaturateOnIntegerOverflow=on  InputSameDT=on
  Switch5 : Switch  Threshold=40  SaturateOnIntegerOverflow=on  InputSameDT=on
  Switch7 : Switch  Threshold=120  SaturateOnIntegerOverflow=on  InputSameDT=on
  Switch8 : Switch  Threshold=40  SaturateOnIntegerOverflow=on  InputSameDT=on
  my1 noise : UniformRandomNumber  Minimum=-rate_noise_my1  Maximum=rate_noise_my1  Seed=seed  SampleTime=0
  "real and false level " : Scope
  Out5 : Outport  InitialOutput=0
  Out1 : Outport  Port=2  InitialOutput=0
  Out2 : Outport  Port=3  InitialOutput=0
  wires:
  Clock2/1 -> Switch1/2, Switch4/2
  Constant1/1 -> Switch1/1
  Switch1/1 -> Switch4/3
  Switch4/1 -> Commande vanne 2/2
  In1/1 -> Switch1/3, Switch4/1, Commande vanne 2/1
  Commande vanne 2/1 -> Sum6/1
  my1 noise/1 -> Sum6/2
  Sum6/1 -> Out1/1, Mux/2, Sum1/1
  Clock1/1 -> Switch5/2, Switch3/2
  Constant4/1 -> Switch5/1
  Constant/1 -> Switch5/3, Switch3/1
  Switch5/1 -> Switch3/3
  Switch3/1 -> Commande vanne 1/1
  Constant5/1 -> Commande vanne 1/2
  Integrator2/1 -> Gain/1
  Mux/1 -> "real and false level "/1
  Commande vanne 1/1 -> Integrator2/1
  Gain/1 -> Sum1/2
  Clock4/1 -> Switch8/2, Switch7/2
  Constant7/1 -> Switch8/1
  Constant6/1 -> Switch8/3, Switch7/1
  Switch8/1 -> Switch7/3
  Switch7/1 -> Commande vanne 4/1
  Constant8/1 -> Commande vanne 4/2
  Integrator1/1 -> Stolen Volume/1, Out2/1
  Commande vanne 4/1 -> Integrator1/1
  Sum1/1 -> Mux/1, Out5/1

== system CHEM_FULL_BENCHMARK/T1 semi hidden long theft/Process/Subsystem8 ==
  note: SIMULATION OF TANK T2
  note: Faultless mode
  note: Faulty mode
      | water leak
  Qvo : Inport
  Qvb : Inport  Port=2
  Clock2 : Clock
  Commande vanne 2 : ManualSwitch  CurrentSetting=0
  Constant : Constant  Value=0
  Constant1 : Constant  Value=Qf2
  Constant2 : Constant  Value=0
  Gain : Gain  Gain=1/A2  SaturateOnIntegerOverflow=on  OutDataTypeStr=Inherit: Same as input  ParamDataTypeStr=Inherit: Same as input
  Integrator2 : Integrator  InitialCondition=h2c_0
  Saturation1 : Saturate  UpperLimit=h2max  LowerLimit=0  LinearizeAsGain=off
  Sum2 : Sum  Inputs=-+-  SaturateOnIntegerOverflow=on  InputSameDT=on  OutDataTypeStr=Inherit: Same as first input
  Switch1 : Switch  Threshold=120  SaturateOnIntegerOverflow=on  InputSameDT=on
  Switch4 : Switch  Threshold=40  SaturateOnIntegerOverflow=on  InputSameDT=on
  y2 : Outport  InitialOutput=0
  wires:
  Qvb/1 -> Sum2/2
  Qvo/1 -> Sum2/1
  Sum2/1 -> Gain/1
  Gain/1 -> Integrator2/1
  Clock2/1 -> Switch4/2, Switch1/2
  Constant1/1 -> Switch4/1
  Constant/1 -> Switch4/3, Switch1/1
  Switch4/1 -> Switch1/3
  Commande vanne 2/1 -> Sum2/3
  Switch1/1 -> Commande vanne 2/1
  Constant2/1 -> Commande vanne 2/2
  Integrator2/1 -> Saturation1/1
  Saturation1/1 -> y2/1

== system CHEM_FULL_BENCHMARK/T1 semi hidden long theft/Process/Subsystem9 ==
  Subsystem1 : Subsystem
      mask Display: disp('Set \nvalve  V2')
  Subsystem12 : Subsystem
      mask Display: disp('Set\n point h1c')
  Out3 : Outport  InitialOutput=0
  Out1 : Outport  Port=2  InitialOutput=0
  wires:
  Subsystem1/1(Out1) -> Out1/1
  Subsystem12/1(Out1) -> Out3/1

== system CHEM_FULL_BENCHMARK/T1 short theft/Process/Subsystem1 ==
  note: TANK T1 SIMULATION
  note: Qf1
  note: Faultless mode
  note: Faulty mode
      | water leak
  Qp : Inport
  Qvb : Inport  Port=2
  Clock2 : Clock
  Constant : Constant  Value=0
  Constant2 : Constant  Value=0
  Gain : Gain  Gain=1/A1  SaturateOnIntegerOverflow=on  OutDataTypeStr=Inherit: Same as input  ParamDataTypeStr=Inherit: Same as input
  Integrator2 : Integrator  InitialCondition=h1c_0
  Saturation1 : Saturate  UpperLimit=h1max  LowerLimit=0  LinearizeAsGain=off
  Selector : ManualSwitch
  Sum2 : Sum  Inputs=+--  SaturateOnIntegerOverflow=on  InputSameDT=on  OutDataTypeStr=Inherit: Same as first input
  Switch1 : Switch  Threshold=80  SaturateOnIntegerOverflow=on  InputSameDT=on
  Switch4 : Switch  Threshold=40  SaturateOnIntegerOverflow=on  InputSameDT=on
  flow leak : Constant  Value=Qf1
  y1 : Outport  InitialOutput=0
  wires:
  Gain/1 -> Integrator2/1
  Sum2/1 -> Gain/1
  Qp/1 -> Sum2/1
  Qvb/1 -> Sum2/2
  Clock2/1 -> Switch4/2, Switch1/2
  flow leak/1 -> Switch4/1
  Constant/1 -> Switch4/3, Switch1/1
  Switch4/1 -> Switch1/3
  Selector/1 -> Sum2/3
  Switch1/1 -> Selector/1
  Constant2/1 -> Selector/2
  Integrator2/1 -> Saturation1/1
  Saturation1/1 -> y1/1

== system CHEM_FULL_BENCHMARK/T1 short theft/Process/Subsystem10 ==
  note: SIMULATION OF THE SENSOR y2
  note: Faultless mode
  note: Faulty mode
  note: Faultless mode
  note: Faulty mode
      | water leak
  note: Faultless mode
  note: Faulty mode
      | water leak
  y2 : Inport
  Clock1 : Clock
  Clock2 : Clock
  Clock3 : Clock
  Commande vanne 1 : ManualSwitch  CurrentSetting=0
  Commande vanne 2 : ManualSwitch
  Commande vanne 3 : ManualSwitch  CurrentSetting=0
  Constant{,1,3..4,6} (5 alike) : Constant  Value=0
  Constant2 : Constant  Value=Qf2/2
  Constant5 : Constant  Value=Qf2
  Gain : Gain  Gain=1/A2  SaturateOnIntegerOverflow=on  OutDataTypeStr=Inherit: Same as input  ParamDataTypeStr=Inherit: Same as input
  Integrator1 : Integrator
  Integrator2 : Integrator
  Mux : Mux  Inputs=2
  Stolen Volume : Scope
  Sum1 : Sum  SaturateOnIntegerOverflow=on  InputSameDT=on  OutDataTypeStr=Inherit: Same as first input
  Sum6 : Sum  SaturateOnIntegerOverflow=on  InputSameDT=on  OutDataTypeStr=Inherit: Same as first input
  Switch1 : Switch  Threshold=40  SaturateOnIntegerOverflow=on  InputSameDT=on
  Switch2 : Switch  Threshold=120  SaturateOnIntegerOverflow=on  InputSameDT=on
  Switch3 : Switch  Threshold=40  SaturateOnIntegerOverflow=on  InputSameDT=on
  Switch4 : Switch  Threshold=120  SaturateOnIntegerOverflow=on  InputSameDT=on
  Switch5 : Switch  Threshold=120  SaturateOnIntegerOverflow=on  InputSameDT=on
  Switch6 : Switch  Threshold=40  SaturateOnIntegerOverflow=on  InputSameDT=on
  my2 noise : UniformRandomNumber  Minimum=-rate_noise_my2  Maximum=rate_noise_my2  Seed=seed  SampleTime=0
  "real and false level " : Scope
  my2 : Outport  InitialOutput=0
  yy2 : Outport  Port=2  InitialOutput=0
  vol2 : Outport  Port=3  InitialOutput=0
  wires:
  my2 noise/1 -> Sum6/2
  Commande vanne 2/1 -> Sum6/1
  y2/1 -> Commande vanne 2/1, Switch1/3, Switch4/1
  Switch4/1 -> Commande vanne 2/2
  Switch1/1 -> Switch4/3
  Constant1/1 -> Switch1/1
  Clock2/1 -> Switch4/2, Switch1/2
  Clock1/1 -> Switch3/2, Switch2/2
  Constant2/1 -> Switch3/1
  Constant/1 -> Switch3/3, Switch2/1
  Switch3/1 -> Switch2/3
  Switch2/1 -> Commande vanne 1/1
  Constant3/1 -> Commande vanne 1/2
  Sum6/1 -> yy2/1, Mux/2, Sum1/1
  Sum1/1 -> Mux/1, my2/1
  Integrator2/1 -> Gain/1
  Mux/1 -> "real and false level "/1
  Commande vanne 1/1 -> Integrator2/1
  Gain/1 -> Sum1/2
  Clock3/1 -> Switch6/2, Switch5/2
  Constant5/1 -> Switch6/1
  Constant4/1 -> Switch6/3, Switch5/1
  Switch6/1 -> Switch5/3
  Switch5/1 -> Commande vanne 3/1
  Constant6/1 -> Commande vanne 3/2
  Integrator1/1 -> vol2/1, Stolen Volume/1
  Commande vanne 3/1 -> Integrator1/1
